simulink model "Motor_test"  (R2016b)
settings: Solver=FixedStepAuto  StartTime=0.0  StopTime=rpm_max*1.5  FixedStep=100  RelTol=1e-3
values from neighbouring files (symbols this model uses):
  motor_eff = 0.91    [Init_PI_reg.m]    (also in Initial_test.m; battery_test_res.mat; body_test_res.mat; motor_test_res.mat)
  power_max = 160e3    (= 160000)    [Init_PI_reg.m]    (also in Initial_test.m; battery_test_res.mat; body_test_res.mat; motor_test_res.mat)
  rpm_max = 11688    [Init_PI_reg.m]    (also in Initial_test.m; battery_test_res.mat; body_test_res.mat; motor_test_res.mat)
  torque_max = 300    [Init_PI_reg.m]    (also in Initial_test.m; battery_test_res.mat; body_test_res.mat; motor_test_res.mat)
libraries: simulink x1
settings Model: Creator=a037702  LastModifiedBy=a037702

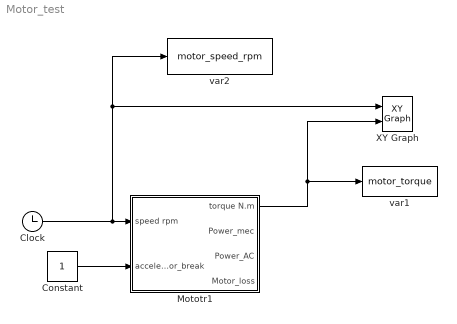
== system Motor_test ==
  Clock : Clock
  Constant : Constant
  Mototr1 : Subsystem
  XY Graph : simulink/Sinks/XY Graph  xmin=-inf  xmax=inf  ymin=-inf  ymax=inf  st=-1
  var1 : ToWorkspace  VariableName=motor_torque  SaveFormat=Structure With Time  SampleTime=-1
      settings: Save2DSignal=2-D array (concatenate along first dimension)
  var2 : ToWorkspace  VariableName=motor_speed_rpm  SaveFormat=Structure With Time  SampleTime=-1
      settings: Save2DSignal=2-D array (concatenate along first dimension)
  wires:
  Mototr1/1(torque N.m) -> XY Graph/2, var1/1
  Clock/1 -> Mototr1/1(speed rpm), XY Graph/1, var2/1
  Constant/1 -> Mototr1/2(accelerator_break)

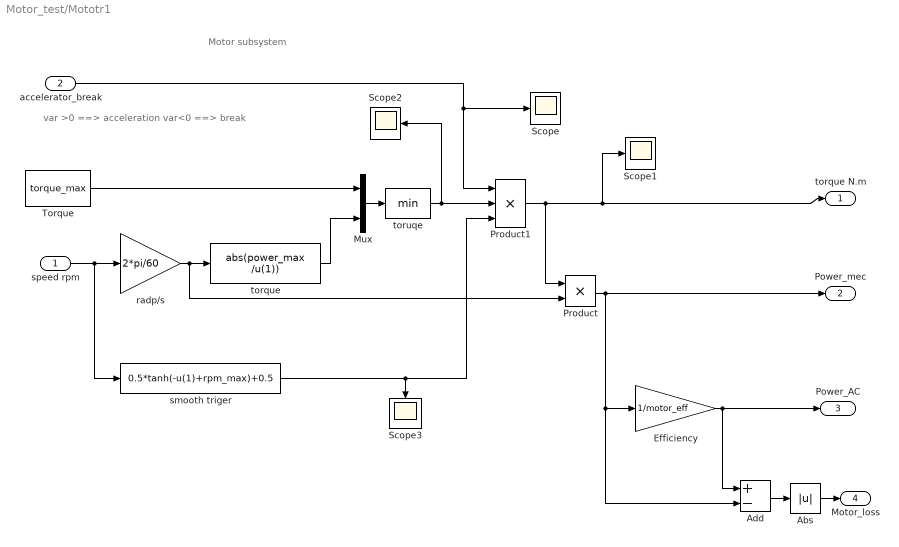
== system Motor_test/Mototr1 ==
  note: var >0 ==> acceleration var<0 ==> break
  note: Motor subsystem
  speed rpm : Inport
  accelerator_break : Inport  Port=2
  Abs : Abs
  Add : Sum  Inputs=+-
  Efficiency : Gain  Gain=1/motor_eff
  Mux : Mux  Inputs=2
  Product : Product
  Product1 : Product  Inputs=3
  Scope{,1..3} (4 alike) : Scope
  Torque : Constant  Value=torque_max
  radp/s : Gain  Gain=2*pi/60
  smooth triger : Fcn  Expr=0.5*tanh(-u(1)+rpm_max)+0.5
  torque : Fcn  Expr=abs(power_max /u(1))
  toruqe : MinMax
  torque N.m : Outport
  Power_mec : Outport  Port=2
  Power_AC : Outport  Port=3
  Motor_loss : Outport  Port=4
  wires:
  Product1/1 -> Product/1, Scope1/1, torque N.m/1
  Mux/1 -> toruqe/1
  Torque/1 -> Mux/1
  radp/s/1 -> Product/2, torque/1
  torque/1 -> Mux/2
  speed rpm/1 -> smooth triger/1, radp/s/1
  Product/1 -> Add/2, Efficiency/1, Power_mec/1
  Efficiency/1 -> Add/1, Power_AC/1
  Add/1 -> Abs/1
  toruqe/1 -> Product1/2, Scope2/1
  accelerator_break/1 -> Scope/1, Product1/1
  Abs/1 -> Motor_loss/1
  smooth triger/1 -> Product1/3, Scope3/1
